simulink model "week3_2016741077_imseyeong_simul"  (R2021a)
settings: Solver=VariableStepAuto  StartTime=0.0  StopTime=10.0  RelTol=1e-3
values from neighbouring files (symbols this model uses):
  B_load = J_load/t    (= 9.65003047429)    [week3_2016741077_imseyeong.m]
  Beq = bm + k*bg    (= 0.00264630474582)    [week3_2016741077_imseyeong.m]
  bm = Jm/t    (= 0.00264627659574)    [week3_2016741077_imseyeong.m]
  J_load = m_bar*(L_bar^2 + 0.25*H_bar^2)/3 + 0.5*m_circle*R_circle^2 + m_circle*L_bar^2    (= 0.0362841145833)    [week3_2016741077_imseyeong.m]
  Jeq = Jm + k*Jg    (= 9.9501058443e-06)    [week3_2016741077_imseyeong.m]
  Jm = 99.5*10^-2*10^-2*10^-3    (= 9.95e-06)    [week3_2016741077_imseyeong.m]
  k = 1/a*(1/n)^2    (= 0.000211688597605)    [week3_2016741077_imseyeong.m]
  Ke = 68.3*10^-3    (= 0.0683)    [week3_2016741077_imseyeong.m]
  Kt = 68.3*10^-3    (= 0.0683)    [week3_2016741077_imseyeong.m]
  La = 0.658*10^-3    (= 0.000658)    [week3_2016741077_imseyeong.m]
  n = 81    [week3_2016741077_imseyeong.m]
  Ra = 1.76    [week3_2016741077_imseyeong.m]
  Va = 48    [week3_2016741077_imseyeong.m]
settings Model: Creator=syl12  LastModifiedBy=syl12

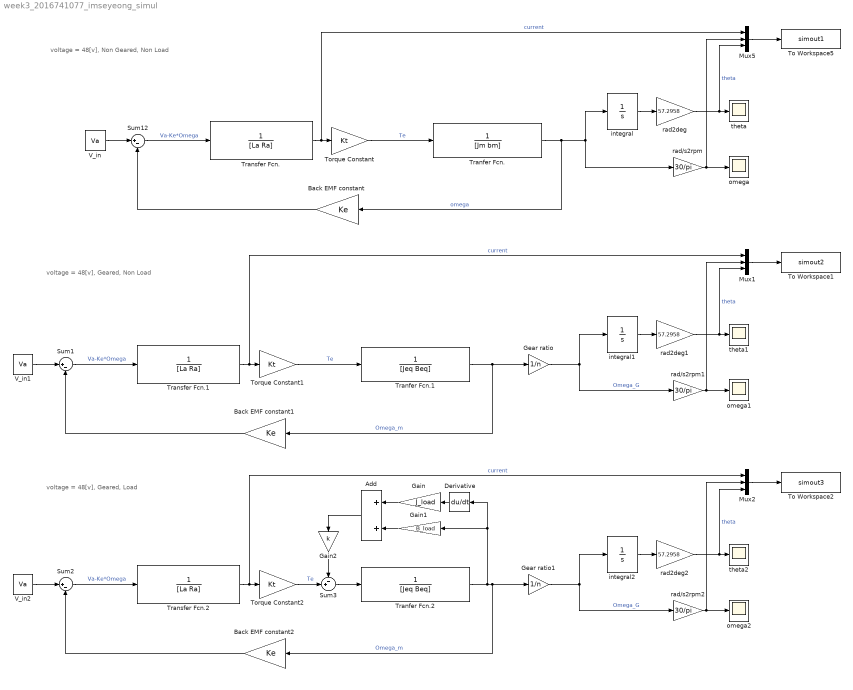
== system week3_2016741077_imseyeong_simul ==
  note: voltage = 48[v], Non Geared, Non Load
  note: voltage = 48[v], Geared, Non Load
  note: voltage = 48[v], Geared, Load
  Add : Sum
  Back EMF constant : Gain  Gain=Ke
  Back EMF constant1 : Gain  Gain=Ke
  Back EMF constant2 : Gain  Gain=Ke
  Derivative : Derivative
  Gain : Gain  Gain=J_load
  Gain1 : Gain  Gain=B_load
  Gain2 : Gain  Gain=k
  Gear ratio : Gain  Gain=1/n
  Gear ratio1 : Gain  Gain=1/n
  Mux1 : Mux  Inputs=3
  Mux2 : Mux  Inputs=3
  Mux5 : Mux  Inputs=3
  Sum1 : Sum  Inputs=|+-
  Sum12 : Sum  Inputs=|+-
  Sum2 : Sum  Inputs=|+-
  Sum3 : Sum  Inputs=-+|
  To Workspace1 : ToWorkspace  VariableName=simout2  SaveFormat=Structure With Time  SampleTime=-1
  To Workspace2 : ToWorkspace  VariableName=simout3  SaveFormat=Structure With Time  SampleTime=-1
  To Workspace5 : ToWorkspace  VariableName=simout1  SaveFormat=Structure With Time  SampleTime=-1
  Torque Constant : Gain  Gain=Kt
  Torque Constant1 : Gain  Gain=Kt
  Torque Constant2 : Gain  Gain=Kt
  Tranfer Fcn. : TransferFcn  Denominator=[Jm bm]
  Tranfer Fcn.1 : TransferFcn  Denominator=[Jeq Beq]
  Tranfer Fcn.2 : TransferFcn  Denominator=[Jeq Beq]
  Transfer Fcn. : TransferFcn  Denominator=[La Ra]
  Transfer Fcn.1 : TransferFcn  Denominator=[La Ra]
  Transfer Fcn.2 : TransferFcn  Denominator=[La Ra]
  V_in : Constant  Value=Va
  V_in1 : Constant  Value=Va
  V_in2 : Constant  Value=Va
  integral : TransferFcn  Denominator=[1 0]
  integral1 : TransferFcn  Denominator=[1 0]
  integral2 : TransferFcn  Denominator=[1 0]
  omega : Scope
  omega1 : Scope
  omega2 : Scope
  rad/s2rpm : Gain  Gain=30/pi
  rad/s2rpm1 : Gain  Gain=30/pi
  rad/s2rpm2 : Gain  Gain=30/pi
  rad2deg : Gain  Gain=57.2958
  rad2deg1 : Gain  Gain=57.2958
  rad2deg2 : Gain  Gain=57.2958
  theta : Scope
  theta1 : Scope
  theta2 : Scope
  wires:
  rad2deg/1 -> Mux5/3, theta/1  "theta"
  Back EMF constant/1 -> Sum12/2
  Tranfer Fcn./1 -> rad/s2rpm/1, integral/1, Back EMF constant/1  "omega"
  Mux5/1 -> To Workspace5/1
  V_in/1 -> Sum12/1
  Transfer Fcn./1 -> Mux5/1, Torque Constant/1  "current"
  integral/1 -> rad2deg/1
  Sum12/1 -> Transfer Fcn./1  "Va-Ke*Omega"
  Torque Constant/1 -> Tranfer Fcn./1  "Te"
  rad/s2rpm/1 -> Mux5/2, omega/1
  rad2deg1/1 -> Mux1/3, theta1/1  "theta"
  Sum1/1 -> Transfer Fcn.1/1  "Va-Ke*Omega"
  integral1/1 -> rad2deg1/1
  Transfer Fcn.1/1 -> Mux1/1, Torque Constant1/1  "current"
  V_in1/1 -> Sum1/1
  Mux1/1 -> To Workspace1/1
  Tranfer Fcn.1/1 -> Gear ratio/1, Back EMF constant1/1  "Omega_m"
  rad/s2rpm1/1 -> Mux1/2, omega1/1
  Torque Constant1/1 -> Tranfer Fcn.1/1  "Te"
  Back EMF constant1/1 -> Sum1/2
  Gear ratio/1 -> rad/s2rpm1/1, integral1/1  "Omega_G"
  Gear ratio1/1 -> rad/s2rpm2/1, integral2/1  "Omega_G"
  rad2deg2/1 -> Mux2/3, theta2/1  "theta"
  rad/s2rpm2/1 -> Mux2/2, omega2/1
  Back EMF constant2/1 -> Sum2/2
  Mux2/1 -> To Workspace2/1
  Tranfer Fcn.2/1 -> Gain1/1, Derivative/1, Gear ratio1/1, Back EMF constant2/1  "Omega_m"
  integral2/1 -> rad2deg2/1
  Sum2/1 -> Transfer Fcn.2/1  "Va-Ke*Omega"
  V_in2/1 -> Sum2/1
  Transfer Fcn.2/1 -> Mux2/1, Torque Constant2/1  "current"
  Gain1/1 -> Add/2
  Add/1 -> Gain2/1
  Derivative/1 -> Gain/1
  Gain/1 -> Add/1
  Gain2/1 -> Sum3/1
  Torque Constant2/1 -> Sum3/2  "Te"
  Sum3/1 -> Tranfer Fcn.2/1
